simulink model "Linear_model_FSFA"  (R2018b)
settings: Solver=VariableStepAuto  StartTime=0.0  StopTime=500  RelTol=1e-3
values from neighbouring files (symbols this model uses):
  a2 = input(12)    [Nonlinear_model.m]    (also in linear_model.m; linear_model_error.m; trailer_constants.m = 4.98)
  Am = [-0.5 0 0 0 0 0 0 0 ... (first row only)    [Dynamic_model_articulation.m]
  Ap = A    [Dynamic_model_articulation.m]    (also in articulation.m = -1*M_inv*K/u)
  B1 = [0,B1(1),0,B1(2),0,B1(3),0,B1(4)]'    [articulation1.m]
  B2 = [0,B2(1),0,B2(2),0,B2(3),0,B2(4)]'    [articulation1.m]
  Bm = [1;0;0;0]    [Dynamic_model_articulation.m]
  Bp = B2    [Dynamic_model_articulation.m]    (also in articulation.m = M_inv*delta)
  constants = [C1 C2 C3 m1 m2 I1 I2 a1 l1 h1 b1 a2 l2 Vx]    [Dynamic_model_articulation.m]
  h1 = input(10)    [Nonlinear_model.m]    (also in linear_model.m; linear_model_error.m; truck_constants.m = 1.1)
  K = place(A,B1,Poles)    [FullStateFeedback.m]    (also in articulation.m = [(C+C3),     (Cs1-C3*(h1+l2)+(m1+m2)*u^2),    (-C3*l2),    (; articulation1.m = [(C+C3),     (Cs1-C3*(h1+l2)+(m1+m2)*u^2),    (-C3*l2),    (; linear_model.m = -1/u*K*x_bar; linear_model_error.m = -1/u*K*x_bar)
  N = 79.8589    [Dynamic_model_articulation.m]
  N2 = 2    [Dynamic_model_articulation.m]
  Pm = lyap(Am,Q)    [Dynamic_model_articulation.m]
  Vx = 20    [Dynamic_model_articulation.m]
settings Model: Creator=kevingasik  LastModifiedBy=kevingasik

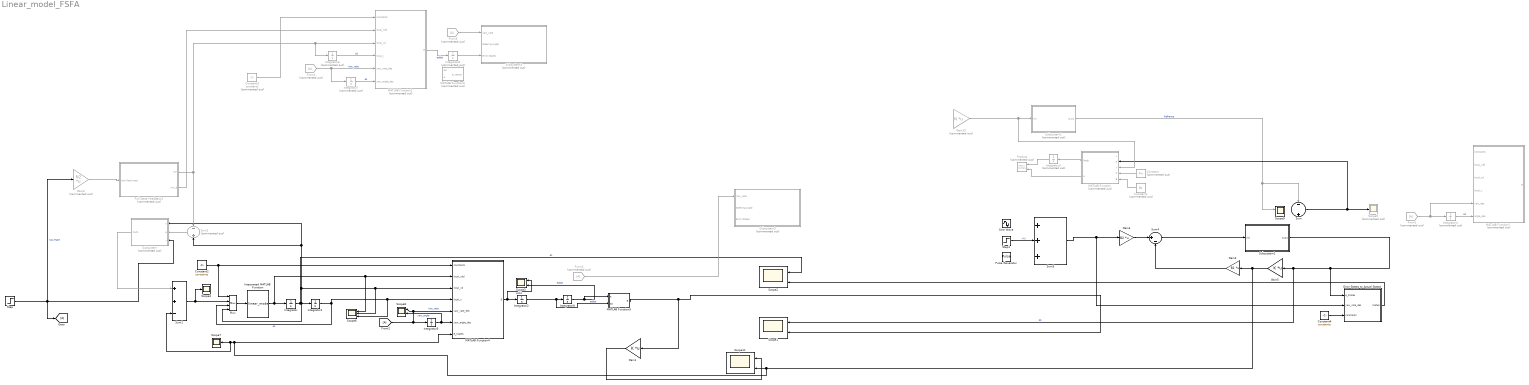
== system Linear_model_FSFA ==
  Constant : Constant  Commented=on  Value=Pm  VectorParams1D=off
  Constant1 : Constant  Commented=on  Value=Bp  VectorParams1D=off
  Constant2 : Constant  Value=constants
  Constant3 : Constant  Commented=on  Value=constants
  Constant4 : Constant  Value=constants
  Error States to Actual Statse : MATLAB Function  TreatAsAtomicUnit=on
  From{1,3..5} (4 alike) : From  Commented=on
  Full State FeedBack2 : Subsystem  Commented=on
  Gain1 : Gain  Gain=K  Multiplication=Matrix(K*u)
  Gain10 : Gain  Commented=on  Gain=N  Multiplication=Matrix(K*u)
  Gain3 : Gain  Gain=B1  Multiplication=Matrix(K*u)
  Gain4 : Gain  Gain=B2  Multiplication=Matrix(K*u)
  Gain5 : Gain  Gain=K  Multiplication=Matrix(K*u)
  Gain6 : Gain  Commented=on  Gain=N2  Multiplication=Matrix(K*u)
  Integrator : Integrator  InitialCondition=[0 0 0 0]
  Integrator1 : Integrator  InitialCondition=[0 0 0 0]
  Integrator2 : Integrator
  Integrator{3..4,6..8} (5 alike) : Integrator  Commented=on
  Integrator5 : Integrator
  Integrator9 : Integrator
  Interpreted MATLAB Function : MATLABFcn  MATLABFcn=linear_model
  MATLAB Function : MATLAB Function  Commented=on  TreatAsAtomicUnit=on
  MATLAB Function1 : MATLAB Function  Commented=on  TreatAsAtomicUnit=on
  MATLAB Function2 : MATLAB Function  Commented=on  TreatAsAtomicUnit=on
  MATLAB Function3 : MATLAB Function  Commented=on  TreatAsAtomicUnit=on
  MATLAB Function4 : MATLAB Function  TreatAsAtomicUnit=on
  MATLAB Function5 : MATLAB Function  TreatAsAtomicUnit=on
  Mux : Mux
  Product : Product  Commented=on  Multiplication=Matrix(*)
  Pulse Generator : DiscretePulseGenerator  PulseType=Time based  Amplitude=0.01  Period=10  PulseWidth=50
  Scope{1..3,8..9,11} (6 alike) : Scope  NumInputPorts=2
  Scope4 : Scope
  Scope5 : Scope  Commented=on
  Scope6 : Scope  NumInputPorts=3
  Scope7 : Scope
  Sine Wave : Sin  Amplitude=0.1  SampleTime=0
  Step : Step  Time=0  After=0.5*pi/180  SampleTime=0
  Step1 : Step  Time=0  After=0.5*pi/180  SampleTime=0
  Subsystem : Subsystem  Commented=on
  Subsystem1 : Subsystem  Commented=on
  Subsystem2 : Subsystem
  Subsystem3 : Subsystem  Commented=on
  Subsystem4 : Subsystem  Commented=on
  Sum : Sum  Inputs=-+
  Sum1 : Sum  Inputs=++-
  Sum2 : Sum  Commented=on  Inputs=-+
  Sum4 : Sum  Inputs=|+-
  Sum5 : Sum  Inputs=+++
  wires:
  Integrator/1 -> Integrator1/1, Mux/4, Sum2/2, Subsystem/1(x), Scope6/2, MATLAB Function4/3(local_xd), Scope2/1  "e1"
  Interpreted MATLAB Function/1 -> Scope6/1, MATLAB Function4/2(local_xdd), Integrator/1
  Mux/1 -> Interpreted MATLAB Function/1
  Integrator1/1 -> Mux/3, Scope6/3, MATLAB Function4/4(local_x)  "e1"
  [A] -> MATLAB Function4/5(yaw_rate_des), Scope8/1, Integrator5/1  "Yaw_rate"
  Integrator5/1 -> Scope8/2, MATLAB Function4/6(yaw_angle_des)  "yaw_angle"
  Constant2/1 -> Mux/1, MATLAB Function4/1(constants)
  Step/1 -> Subsystem/3(r), [A], Gain6/1  "Yaw Rate"
  Sum2/1 -> Subsystem/2(e)
  Full State FeedBack2/1(Xm) -> Sum2/1, Integrator6/1, MATLAB Function2/3(local_xd)
  Gain6/1 -> Full State FeedBack2/1(Yaw Rate Input)
  Sum1/1 -> Mux/2, Scope4/1
  Subsystem/1(Out1) -> Sum1/1
  Subsystem1/1(Out1) -> Scope9/1, Sum/1  "Refrence"
  Constant1/1 -> MATLAB Function/5(B)
  Sum5/1 -> Error States to Actual Statse/2(yaw_rate_des), Gain4/1
  Sum/1 -> Scope5/1, MATLAB Function/2(e)
  Integrator3/1 -> Product/1
  Gain10/1 -> MATLAB Function/3(r), Subsystem1/1(r(t))
  MATLAB Function/1(Nadp) -> Integrator3/1
  Sum4/1 -> Subsystem2/1(r(t))
  Constant/1 -> MATLAB Function/4(P)
  MATLAB Function/2(w) -> Product/2
  Step1/1 -> Sum5/2  "r(t)"
  ? -> MATLAB Function1/2(local_xdd)
  ? -> MATLAB Function1/1(constants)
  Subsystem2/1(Out1) -> Error States to Actual Statse/1(e_states), Scope1/1, Gain5/1  "SS"
  ? -> MATLAB Function1/4(local_x)  "e1"
  From1/1 -> Integrator4/1, MATLAB Function1/5(yaw_des)
  Integrator4/1 -> MATLAB Function1/6(angle_des)  "e1"
  MATLAB Function4/1(E) -> Scope3/1, Integrator2/1  "eddot"
  From3/1 -> Subsystem3/1(Yaw_rate)
  Constant3/1 -> MATLAB Function2/1(constants)
  Full State FeedBack2/2(Xm_d) -> MATLAB Function2/2(local_xdd)
  Integrator6/1 -> MATLAB Function2/4(local_x)  "e1"
  From4/1 -> Integrator7/1, MATLAB Function2/5(yaw_rate_des)  "Yaw_rate"
  Integrator7/1 -> MATLAB Function2/6(yaw_angle_des)  "e1"
  MATLAB Function2/1(E) -> Integrator8/1  "eddot"
  From5/1 -> Subsystem4/1(Yaw_rate)
  Integrator8/1 -> Subsystem4/3(Error States)
  Gain3/1 -> Sum4/2
  Gain4/1 -> Sum4/1
  Constant4/1 -> Error States to Actual Statse/3(constants)
  Error States to Actual Statse/1(states) -> Scope2/2
  Integrator2/1 -> MATLAB Function5/2(ed), Integrator9/1  "eddot"
  MATLAB Function5/1(E) -> Scope1/2, Gain1/1
  Integrator9/1 -> MATLAB Function5/1(e), Scope3/2  "eddot"
  Gain5/1 -> MATLAB Function4/7(E_states), Sum1/3, Scope7/1, Scope11/2, Gain3/1
  Gain1/1 -> Scope11/1

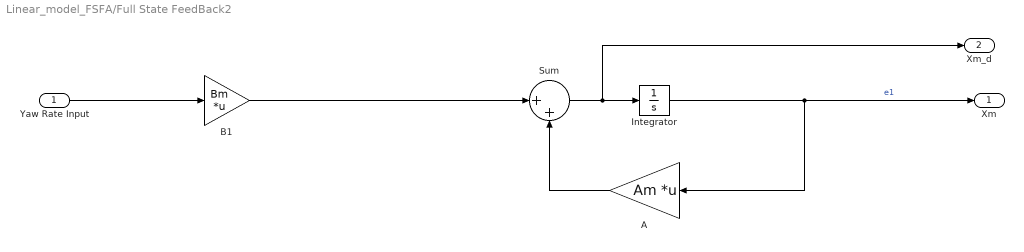
== system Linear_model_FSFA/Full State FeedBack2 ==
  Yaw Rate Input : Inport
  A : Gain  Gain=Am  Multiplication=Matrix(K*u)
  B1 : Gain  Gain=Bm  Multiplication=Matrix(K*u)
  Integrator : Integrator
  Sum : Sum  Inputs=|++
  Xm : Outport
  Xm_d : Outport  Port=2
  wires:
  Sum/1 -> Xm_d/1, Integrator/1
  A/1 -> Sum/2
  Integrator/1 -> Xm/1, A/1  "e1"
  Yaw Rate Input/1 -> B1/1
  B1/1 -> Sum/1

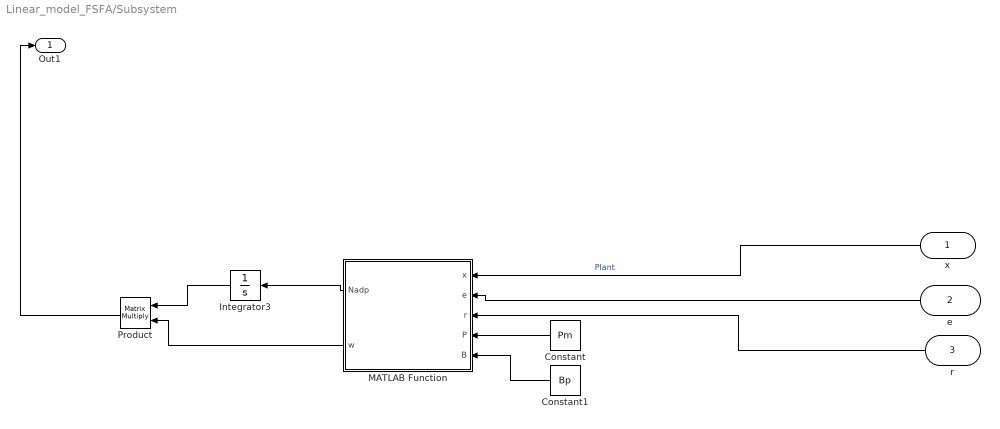
== system Linear_model_FSFA/Subsystem ==
  x : Inport
  e : Inport  Port=2
  r : Inport  Port=3
  Constant : Constant  Value=Pm  VectorParams1D=off
  Constant1 : Constant  Value=Bp  VectorParams1D=off
  Integrator3 : Integrator
  MATLAB Function : MATLAB Function  TreatAsAtomicUnit=on
  Product : Product  Multiplication=Matrix(*)
  Out1 : Outport
  wires:
  r/1 -> MATLAB Function/3(r)
  MATLAB Function/2(w) -> Product/2
  Constant/1 -> MATLAB Function/4(P)
  x/1 -> MATLAB Function/1(x)  "Plant"
  Integrator3/1 -> Product/1
  Product/1 -> Out1/1
  MATLAB Function/1(Nadp) -> Integrator3/1
  e/1 -> MATLAB Function/2(e)
  Constant1/1 -> MATLAB Function/5(B)

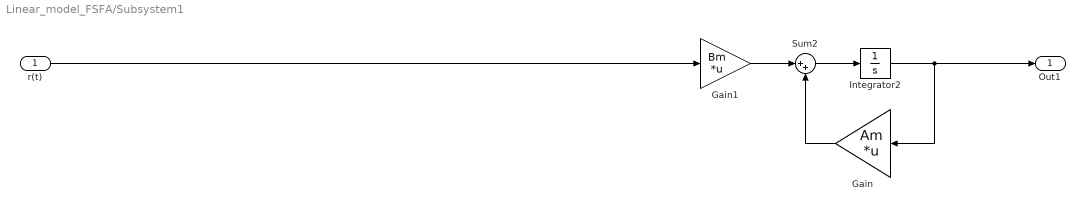
== system Linear_model_FSFA/Subsystem1 ==
  r(t) : Inport
  Gain : Gain  Gain=Am  Multiplication=Matrix(K*u)
  Gain1 : Gain  Gain=Bm  Multiplication=Matrix(K*u)
  Integrator2 : Integrator  InitialCondition=[0 0 0 0]
  Sum2 : Sum  Inputs=|++
  Out1 : Outport
  wires:
  Sum2/1 -> Integrator2/1
  Gain/1 -> Sum2/2
  Gain1/1 -> Sum2/1
  r(t)/1 -> Gain1/1
  Integrator2/1 -> Out1/1, Gain/1

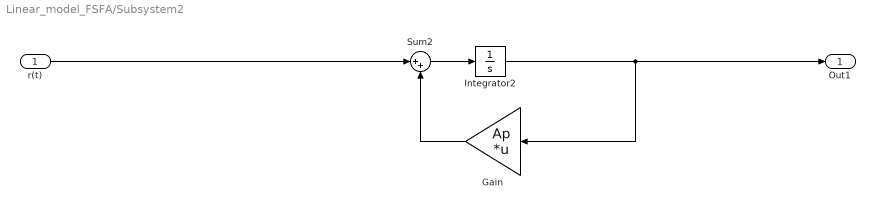
== system Linear_model_FSFA/Subsystem2 ==
  r(t) : Inport
  Gain : Gain  Gain=Ap  Multiplication=Matrix(K*u)
  Integrator2 : Integrator
  Sum2 : Sum  Inputs=|++
  Out1 : Outport
  wires:
  Sum2/1 -> Integrator2/1
  r(t)/1 -> Sum2/1
  Integrator2/1 -> Out1/1, Gain/1
  Gain/1 -> Sum2/2

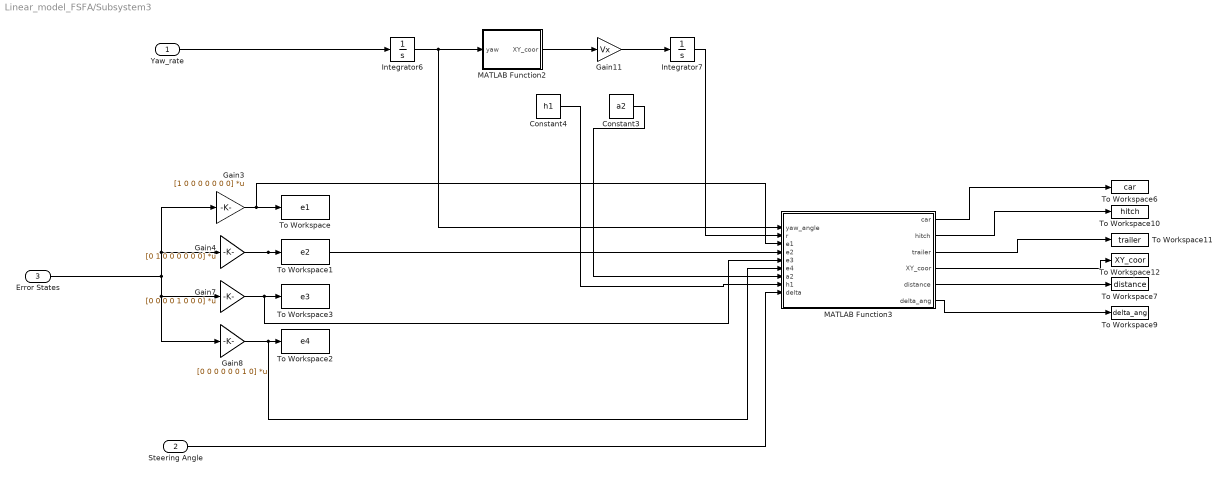
== system Linear_model_FSFA/Subsystem3 ==
  Yaw_rate : Inport
  Steering Angle : Inport  Port=2
  Error States : Inport  Port=3
  Constant3 : Constant  Value=a2
  Constant4 : Constant  Value=h1
  Gain11 : Gain  Gain=Vx
  Gain3 : Gain  Gain=[1 0 0 0 0 0 0 0]  Multiplication=Matrix(K*u)
  Gain4 : Gain  Gain=[0 1 0 0 0 0 0 0]  Multiplication=Matrix(K*u)
  Gain7 : Gain  Gain=[0 0 0 0 1 0 0 0]  Multiplication=Matrix(K*u)
  Gain8 : Gain  Gain=[0 0 0 0 0 0 1 0]  Multiplication=Matrix(K*u)
  Integrator6 : Integrator
  Integrator7 : Integrator
  MATLAB Function2 : MATLAB Function  TreatAsAtomicUnit=on
  MATLAB Function3 : MATLAB Function  TreatAsAtomicUnit=on
  To Workspace : ToWorkspace  VariableName=e1  SampleTime=-1
  To Workspace1 : ToWorkspace  VariableName=e2  SampleTime=-1
  To Workspace10 : ToWorkspace  VariableName=hitch  SampleTime=-1
      settings: Save2DSignal=2-D array (concatenate along first dimension)
  To Workspace11 : ToWorkspace  VariableName=trailer  SampleTime=-1
      settings: Save2DSignal=2-D array (concatenate along first dimension)
  To Workspace12 : ToWorkspace  VariableName=XY_coor  SampleTime=-1
      settings: Save2DSignal=2-D array (concatenate along first dimension)
  To Workspace2 : ToWorkspace  VariableName=e4  SampleTime=-1
  To Workspace3 : ToWorkspace  VariableName=e3  SampleTime=-1
  To Workspace6 : ToWorkspace  VariableName=car  SampleTime=-1
      settings: Save2DSignal=2-D array (concatenate along first dimension)
  To Workspace7 : ToWorkspace  VariableName=distance  SampleTime=-1
      settings: Save2DSignal=2-D array (concatenate along first dimension)
  To Workspace9 : ToWorkspace  VariableName=delta_ang  SampleTime=-1
      settings: Save2DSignal=2-D array (concatenate along first dimension)
  wires:
  MATLAB Function3/5(distance) -> To Workspace7/1
  Constant4/1 -> MATLAB Function3/8(h1)
  MATLAB Function3/4(XY_coor) -> To Workspace12/1
  Integrator7/1 -> MATLAB Function3/2(r)
  MATLAB Function3/3(trailer) -> To Workspace11/1
  Integrator6/1 -> MATLAB Function3/1(yaw_angle), MATLAB Function2/1(yaw)
  Gain11/1 -> Integrator7/1
  MATLAB Function3/1(car) -> To Workspace6/1
  MATLAB Function2/1(XY_coor) -> Gain11/1
  Steering Angle/1 -> MATLAB Function3/9(delta)
  MATLAB Function3/2(hitch) -> To Workspace10/1
  Gain8/1 -> MATLAB Function3/6(e4), To Workspace2/1
  MATLAB Function3/6(delta_ang) -> To Workspace9/1
  Gain7/1 -> MATLAB Function3/5(e3), To Workspace3/1
  Gain3/1 -> MATLAB Function3/3(e1), To Workspace/1
  Constant3/1 -> MATLAB Function3/7(a2)
  Error States/1 -> Gain8/1, Gain7/1, Gain3/1, Gain4/1
  Yaw_rate/1 -> Integrator6/1
  Gain4/1 -> MATLAB Function3/4(e2), To Workspace1/1

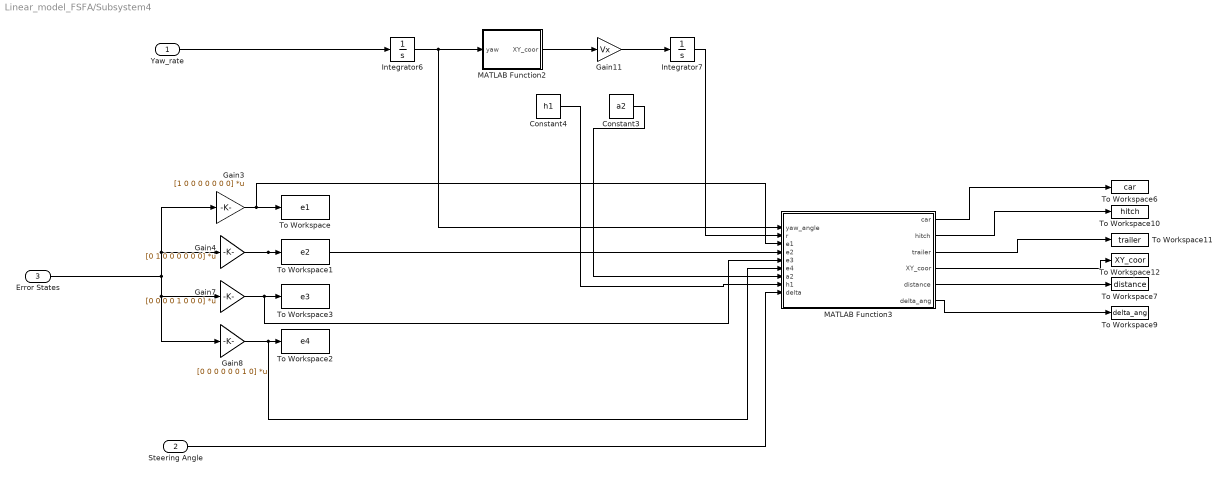
== system Linear_model_FSFA/Subsystem4 ==
  Yaw_rate : Inport
  Steering Angle : Inport  Port=2
  Error States : Inport  Port=3
  Constant3 : Constant  Value=a2
  Constant4 : Constant  Value=h1
  Gain11 : Gain  Gain=Vx
  Gain3 : Gain  Gain=[1 0 0 0 0 0 0 0]  Multiplication=Matrix(K*u)
  Gain4 : Gain  Gain=[0 1 0 0 0 0 0 0]  Multiplication=Matrix(K*u)
  Gain7 : Gain  Gain=[0 0 0 0 1 0 0 0]  Multiplication=Matrix(K*u)
  Gain8 : Gain  Gain=[0 0 0 0 0 0 1 0]  Multiplication=Matrix(K*u)
  Integrator6 : Integrator
  Integrator7 : Integrator
  MATLAB Function2 : MATLAB Function  TreatAsAtomicUnit=on
  MATLAB Function3 : MATLAB Function  TreatAsAtomicUnit=on
  To Workspace : ToWorkspace  VariableName=e1  SampleTime=-1
  To Workspace1 : ToWorkspace  VariableName=e2  SampleTime=-1
  To Workspace10 : ToWorkspace  VariableName=hitch  SampleTime=-1
      settings: Save2DSignal=2-D array (concatenate along first dimension)
  To Workspace11 : ToWorkspace  VariableName=trailer  SampleTime=-1
      settings: Save2DSignal=2-D array (concatenate along first dimension)
  To Workspace12 : ToWorkspace  VariableName=XY_coor  SampleTime=-1
      settings: Save2DSignal=2-D array (concatenate along first dimension)
  To Workspace2 : ToWorkspace  VariableName=e4  SampleTime=-1
  To Workspace3 : ToWorkspace  VariableName=e3  SampleTime=-1
  To Workspace6 : ToWorkspace  VariableName=car  SampleTime=-1
      settings: Save2DSignal=2-D array (concatenate along first dimension)
  To Workspace7 : ToWorkspace  VariableName=distance  SampleTime=-1
      settings: Save2DSignal=2-D array (concatenate along first dimension)
  To Workspace9 : ToWorkspace  VariableName=delta_ang  SampleTime=-1
      settings: Save2DSignal=2-D array (concatenate along first dimension)
  wires:
  MATLAB Function3/5(distance) -> To Workspace7/1
  Constant4/1 -> MATLAB Function3/8(h1)
  MATLAB Function3/4(XY_coor) -> To Workspace12/1
  Integrator7/1 -> MATLAB Function3/2(r)
  MATLAB Function3/3(trailer) -> To Workspace11/1
  Integrator6/1 -> MATLAB Function3/1(yaw_angle), MATLAB Function2/1(yaw)
  Gain11/1 -> Integrator7/1
  MATLAB Function3/1(car) -> To Workspace6/1
  MATLAB Function2/1(XY_coor) -> Gain11/1
  Steering Angle/1 -> MATLAB Function3/9(delta)
  MATLAB Function3/2(hitch) -> To Workspace10/1
  Gain8/1 -> MATLAB Function3/6(e4), To Workspace2/1
  MATLAB Function3/6(delta_ang) -> To Workspace9/1
  Gain7/1 -> MATLAB Function3/5(e3), To Workspace3/1
  Gain3/1 -> MATLAB Function3/3(e1), To Workspace/1
  Constant3/1 -> MATLAB Function3/7(a2)
  Error States/1 -> Gain8/1, Gain7/1, Gain3/1, Gain4/1
  Yaw_rate/1 -> Integrator6/1
  Gain4/1 -> MATLAB Function3/4(e2), To Workspace1/1

== matlab function Linear_model_FSFA/MATLAB Function1 ==
  data: constants input; local_xdd input; local_xd input; local_x input; E output; yaw_des input; angle_des input
function E  = fcn(constants,local_xdd,local_xd,local_x,yaw_des,angle_des)
%% this function takes the local coordinates and converts them into error coordinates
%% to be controlled
E = [0;0;0;0;0;0;0;0];

%% set up constants for equation
Vx = constants(14);
a2 = constants(12);

%% convert local_x to understandable variables
r1 = local_x(2);
yaw = local_x(3);

%% convert x_dot to understandable variables
v1 = local_xd(2);
psi_d = local_xd(3);

%% convert x_ddot to understanable variables
v1d = local_xdd(2);
psi_dd = local_xdd(3);


%% convert local coordinates to fixed coordiates
e1d = v1d + Vx*(yaw-angle_des);
e2d = yaw - angle_des;

e1dd = v1d + Vx*(psi_d-yaw_des);
e2dd = psi_d - yaw_des;


e3d = v1d + Vx*(yaw-angle_des);
e4d = yaw - angle_des;

e3dd = v1d + Vx*(psi_d-yaw_des);
e4dd = psi_d - yaw_des;


E = [e1d;e1dd;e2d;e2dd;e3d;e3dd;e4d;e4dd];

== matlab function Linear_model_FSFA/MATLAB Function ==
  data: x input; Nadp output; e input; r input; P input; w output; B input
function [Nadp,w]   = fcn(x,e,r,P,B)

w = [0;0;0;0;0;0];
Nadp = [0;0;0;0;0;0]';
x = [0; x(2);0;0];
e = [0; e(2);0;0];

%% define learning rate
gr = 2; 
gx = (eye(4))*2;
ydd = 0.1;

%% Thesis paper
w = [x' r 1]';
 
theta_xd = -gx*x*e'*P*B;
theta_d_d = -ydd*e'*P*B;
theta_rd = -gr*e'*P*B;

Nadp = [theta_xd' theta_d_d' theta_rd']

== matlab function Linear_model_FSFA/Subsystem/MATLAB Function ==
  data: x input; Nadp output; e input; r input; P input; w output; B input
function [Nadp,w]   = fcn(x,e,r,P,B)

w = [0;0;0;0;0;0];
Nadp = [0;0;0;0;0;0]';

%x = [0; x(2);x(3);x(4)];
%e = [0; e(2);e(3);e(4)];

%x = [x(1);0;0;0];
%e = [e(1);0;0;0];


%% define learning rate
gr = 0.5; 
gx = [1 0 0 0;
      0 1 0 0;
      0 0 1 0;
      0 0 0 1];

ydd = 0.5;

%% Thesis paper
w = [x' r 1]';
 
theta_xd = -gx*x*e'*P*B;
theta_d_d = -ydd*e'*P*B;
theta_rd = -gr*e'*P*B;

Nadp = [theta_xd' theta_d_d' theta_rd']

== matlab function Linear_model_FSFA/Subsystem3/MATLAB Function2 ==
  data: yaw input; XY_coor output
function XY_coor  = fcn(yaw)

XY_coor = [cos(yaw),sin(yaw)];

== matlab function Linear_model_FSFA/MATLAB Function4 ==
  data: constants input; local_xdd input; local_xd input; local_x input; E output; yaw_rate_des input; yaw_angle_des input; E_states input
function E  = fcn(constants,local_xdd,local_xd,local_x,yaw_rate_des,yaw_angle_des,E_states)
%% this function takes the local coordinates and converts them into error coordinates
%% to be controlled
E = [0;0;0;0];

%% set up constants for equation %%%%%%%%%%%%%%%%%%%%%%%%%%%%%%%%%%%%%%%%%%

C1 = constants(1);
C2 = constants(2);
C3 = constants(3);
m1 = constants(4);
m2 = constants(5);
I1 = constants(6);
I2 = constants(7);
a1 = constants(8);
l1 = constants(9);
h1 = constants(10);
b1 = constants(11);
a2 = constants(12);
l2 = constants(13);
Vx = constants(14);
u = Vx;

C = C1 + C2;
Cs1 = a1*C1 - b1*C2;
Cq1 = sqrt(a1^2*C1 +b1^2*C2);

%% convert local_x to understandable variables %%%%%%%%%%%%%%%%%%%%%%%%%%%%
y1 = local_x(1);
psi = local_x(2);

%% convert x_dot to understandable variables %%%%%%%%%%%%%%%%%%%%%%%%%%%%%%
v1 = local_xd(1);
psi_d = local_xd(2);
phi_d = local_xd(3);
phi = local_xd(4);

%% convert x_ddot to understanable variables %%%%%%%%%%%%%%%%%%%%%%%%%%%%%%
v1d = local_xdd(1);
psi_dd = local_xdd(2);
phi_dd = local_xdd(3);

%% convert local coordinates to global coordiates %%%%%%%%%%%%%%%%%%%%%%%%%
e1d  = v1 + Vx*(psi - yaw_angle_des);
e1dd = v1d + Vx*(psi_d - yaw_rate_des);

e2d  = psi_d - yaw_rate_des;
e2dd = psi_dd;

e3d  = v1 - a2*phi_d + Vx*(psi - yaw_angle_des + phi);
e3dd = v1d - a2*phi_dd + Vx*(psi_d - yaw_rate_des + phi_d);

e4d  = psi_d - yaw_rate_des + phi_d;
e4dd = psi_dd + phi_dd;

eddot_A = [1,   0,          0,      0;
           0,   1,          0,      0;
           1,   0,          -a2,     0; %e3dd = y_dd - a2*phi_dd - Vx(psi_d) + Vx*(phi_d) -Vx*psi_des_d
           0,   1,          1,      0]; %e4dd = psi_dd + phi_dd + psi_desired_dd
             
eddot_B = [0,   Vx,          0,      0;
           0,   0,           0,      0;
           0,   Vx,          Vx,      0;
           0,   0,            0,      0];
       
       
eddot_C = [-Vx,0,-Vx,0]'; % desired yaw rate matrix

E = eddot_A*local_xdd + eddot_B*local_xd + eddot_C*yaw_rate_des;

%E = [e1d,Edd(1),e2d,Edd(2),e3d,Edd(3),e4d,Edd(4)]';
%E = [e1d,e1dd,e2d,e2dd,e3d,e2dd,e4d,e4dd]';

== matlab function Linear_model_FSFA/Subsystem3/MATLAB Function3 ==
  data: yaw_angle input; r input; e1 input; car output; hitch output; trailer output; XY_coor output; e2 input; e3 input; e4 input; a2 input; h1 input; distance output; delta input; delta_ang output
function [car,hitch,trailer,XY_coor,distance,delta_ang] = fcn(yaw_angle,r,e1,e2,e3, e4, a2,h1,delta)
XY_coor = [0 0];
trailer = [0 0];
hitch = [0 0];
car = [0 0];
angle = 0;


%%Transformation matrices from local to global coordinates
Q = [-sin(yaw_angle+e2),cos(yaw_angle+e2)];
R = [-cos(yaw_angle+e2),-sin(yaw_angle+e2)];
T = [-cos(yaw_angle+e4),-sin(yaw_angle+e4)];

%% desired trajectory
X_des = r(1,1);
Y_des = r(1,2);
%X_des2 = r(1,1) - (a2+h1)*cosd(yaw_angle+e2);
%Y_des2 = r(1,2) - (a2+h1)*sind(yaw_angle+e2);
XY_coor = [X_des,Y_des];

%outputting the correct output.
car_x = r(1,1)+ e1*Q(1,1);
car_y = r(1,2)+ e1*Q(1,2);
car = [car_x,car_y];

hitch_x = r(1,1) + e1*Q(1,1) + h1*R(1,1);
hitch_y = r(1,2) + e1*Q(1,2) + h1*R(1,2);
%hitch_a = X_des2 + e3*Q(1,1) - a2*T(1,1);
%hitch_b = Y_des2 + e3*Q(1,2) - a2*T(1,2);
hitch = [hitch_x,hitch_y];


trailer_x = r(1,1)+ (e1)*Q(1,1) + h1*R(1,1) + a2*T(1,1);
trailer_y = r(1,2)+ (e1)*Q(1,2) + h1*R(1,2) + a2*T(1,2);
%trailer_x = X_des2 + e3*Q(1,1);
%trailer_y = Y_des2 + e3*Q(1,2);

distance = sqrt((abs(hitch_x-trailer_x))^2 + abs(hitch_y-trailer_y)^2);
delta_ang = delta + e2 + yaw_angle; 
trailer = [trailer_x,trailer_y];

== matlab function Linear_model_FSFA/MATLAB Function2 ==
  data: constants input; local_xdd input; local_xd input; local_x input; E output; yaw_rate_des input; yaw_angle_des input
function E   = fcn(constants,local_xdd,local_xd,local_x,yaw_rate_des,yaw_angle_des)
%% this function takes the local coordinates and converts them into error coordinates
%% to be controlled
E = [0;0;0;0;0;0;0;0];

%% set up constants for equation %%%%%%%%%%%%%%%%%%%%%%%%%%%%%%%%%%%%%%%%%%

C1 = constants(1);
C2 = constants(2);
C3 = constants(3);
m1 = constants(4);
m2 = constants(5);
I1 = constants(6);
I2 = constants(7);
a1 = constants(8);
l1 = constants(9);
h1 = constants(10);
b1 = constants(11);
a2 = constants(12);
l2 = constants(13);
Vx = constants(14);
u = Vx;

C = C1 + C2;
Cs1 = a1*C1 - b1*C2;
Cq1 = sqrt(a1^2*C1 +b1^2*C2);

%% convert local_x to understandable variables %%%%%%%%%%%%%%%%%%%%%%%%%%%%
y1 = local_x(1);
psi = local_x(2);

%% convert x_dot to understandable variables %%%%%%%%%%%%%%%%%%%%%%%%%%%%%%
v1 = local_xd(1);
psi_d = local_xd(2);
phi_d = local_xd(3);
phi = local_xd(4);

%% convert x_ddot to understanable variables %%%%%%%%%%%%%%%%%%%%%%%%%%%%%%
v1d = local_xdd(1);
psi_dd = local_xdd(2);
phi_dd = local_xdd(3);
phi_d2  = local_xdd(4);
b1 = l1-a1;


%% convert local coordinates to global coordiates %%%%%%%%%%%%%%%%%%%%%%%%%
e1d  = v1 + Vx*(psi - yaw_angle_des);
e1dd = v1d + Vx*(psi_d - yaw_rate_des);

e2d  = psi_d - yaw_rate_des;
e2dd = psi_dd;

e3d  = v1 - a2*phi_d + Vx*(psi - yaw_angle_des + phi);
e3dd = v1d - a2*phi_dd + Vx*(psi_d - yaw_rate_des + phi_d);

e4d  = psi_d - yaw_rate_des + phi_d;
e4dd = psi_dd + phi_dd;

eddot_A = [1,   0,          0,      0;
           0,   1,          0,      0;
           1,   0,          -a2,     0; %e3dd = y_dd - a2*phi_dd - Vx(psi_d) + Vx*(phi_d) -Vx*psi_des_d
           0,   1,          1,      0]; %e4dd = psi_dd + phi_dd + psi_desired_dd
             
eddot_B = [0,   Vx,          0,      0;
           0,   0,           0,      0;
           0,   Vx,          Vx,      0;
           0,   0,            0,      0];
       
       
eddot_C = [-Vx,0,-Vx,0]'; % desired yaw rate matrix

Edd = eddot_A*local_xdd + eddot_B*local_xd + eddot_C*yaw_rate_des;

E = [e1d,Edd(1),e2d,Edd(2),e3d,Edd(3),e4d,Edd(4)]';
E = [e1d,e1dd,e2d,e2dd,e3d,e3dd,e4d,e4dd]';

== matlab function Linear_model_FSFA/Subsystem4/MATLAB Function2 ==
  data: yaw input; XY_coor output
function XY_coor  = fcn(yaw)

XY_coor = [cos(yaw),sin(yaw)];

== matlab function Linear_model_FSFA/Subsystem4/MATLAB Function3 ==
  data: yaw_angle input; r input; e1 input; car output; hitch output; trailer output; XY_coor output; e2 input; e3 input; e4 input; a2 input; h1 input; distance output; delta input; delta_ang output
function [car,hitch,trailer,XY_coor,distance,delta_ang] = fcn(yaw_angle,r,e1,e2,e3, e4, a2,h1,delta)
XY_coor = [0 0];
trailer = [0 0];
hitch = [0 0];
car = [0 0];
angle = 0;


%%Transformation matrices from local to global coordinates
Q = [-sin(yaw_angle+e2),cos(yaw_angle+e2)];
R = [-cos(yaw_angle+e2),-sin(yaw_angle+e2)];
T = [-cos(yaw_angle+e4),-sin(yaw_angle+e4)];

%% desired trajectory
X_des = r(1,1);
Y_des = r(1,2);
%X_des2 = r(1,1) - (a2+h1)*cosd(yaw_angle+e2);
%Y_des2 = r(1,2) - (a2+h1)*sind(yaw_angle+e2);
XY_coor = [X_des,Y_des];

%outputting the correct output.
car_x = r(1,1)+ e1*Q(1,1);
car_y = r(1,2)+ e1*Q(1,2);
car = [car_x,car_y];

hitch_x = r(1,1) + e1*Q(1,1) + h1*R(1,1);
hitch_y = r(1,2) + e1*Q(1,2) + h1*R(1,2);
%hitch_a = X_des2 + e3*Q(1,1) - a2*T(1,1);
%hitch_b = Y_des2 + e3*Q(1,2) - a2*T(1,2);
hitch = [hitch_x,hitch_y];


trailer_x = r(1,1)+ (e1)*Q(1,1) + h1*R(1,1) + a2*T(1,1);
trailer_y = r(1,2)+ (e1)*Q(1,2) + h1*R(1,2) + a2*T(1,2);
%trailer_x = X_des2 + e3*Q(1,1);
%trailer_y = Y_des2 + e3*Q(1,2);

distance = sqrt((abs(hitch_x-trailer_x))^2 + abs(hitch_y-trailer_y)^2);
delta_ang = delta + e2 + yaw_angle; 
trailer = [trailer_x,trailer_y];

== matlab function Linear_model_FSFA/MATLAB Function3 ==
  data: ed input; e_vector output; e input
function e_vector = fcn(ed,e)
e_vector = [0;0;0;0;0;0;0;0];

e_vector = [e(1),ed(1),e(2),ed(2),e(3),ed(3),e(4),ed(4)]';

== matlab function Linear_model_FSFA/Error States to Actual Statse ==
  data: e_states input; yaw_rate_des input; constants input; states output
function states = fcn(e_states,yaw_rate_des,constants)

states = [0;0;0;0];

a2 = constants(12);
u =  constants(14);

e = [e_states(1) e_states(3) e_states(5) e_states(7)]';
ed = [e_states(2) e_states(4) e_states(6) e_states(8)]';


p1 = [1,        0,              0,      0;
      0,        1,              0,      0;
      1/a2,     0,           -1/a2,     0;  
      0,        0,              0,      0];
                
p2 = [0,        -u,      0,      0;
      0,         0,      0,      0;
      0,     -u/a2,      0,   u/a2;
      0,        -1,      0,      1]; %% phi = -e2 + e4
               
p3 = [0;1;0;0]; % \dot \psi desired 

states = p1*ed + p2*e + p3*yaw_rate_des;

== matlab function Linear_model_FSFA/MATLAB Function5 ==
  data: e input; E output; ed input
function E = fcn(e,ed)

E = [0;0;0;0;0;0;0;0];
E = [e(1),ed(1),e(2),ed(2),e(3),ed(3),e(4),ed(4)]';
